simulink model "Constraint"  (R2019a)
settings: Solver=FixedStepAuto  StartTime=0.0  StopTime=100  FixedStep=0.01  RelTol=1e-3
settings Model: Creator=huic  LastModifiedBy=huic
settings SolverCC: MaxConsecutiveZCs=2048

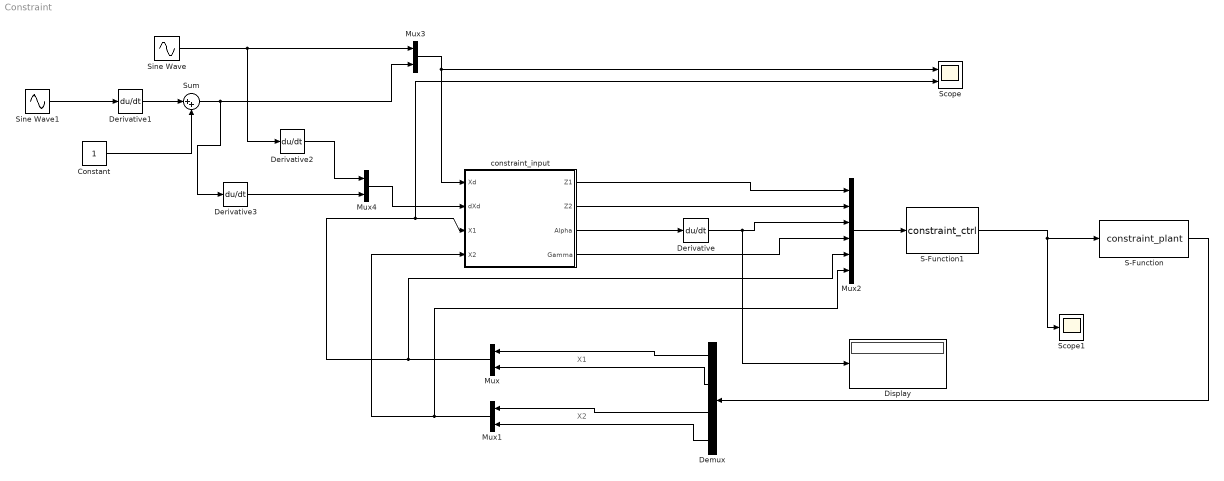
== system Constraint ==
  note: X1
  note: X2
  Constant : Constant
  Demux : Demux
  Derivative{,1..3} (4 alike) : Derivative
  Display : Display
  Mux{,1,3..4} (4 alike) : Mux  Inputs=2
  Mux2 : Mux  Inputs=6
  S-Function : S-Function  FunctionName=constraint_plant  SFunctionDeploymentMode=off  EnableBusSupport=off
  S-Function1 : S-Function  FunctionName=constraint_ctrl  SFunctionDeploymentMode=off  EnableBusSupport=off
  Scope : Scope  NumInputPorts=2
  Scope1 : Scope
  Sine Wave : Sin  SampleTime=0
  Sine Wave1 : Sin  Amplitude=0.3  SampleTime=0
  Sum : Sum  Inputs=|++
  constraint_input : MATLAB Function  TreatAsAtomicUnit=on
  wires:
  S-Function/1 -> Demux/1
  Demux/1 -> Mux/1
  Mux/1 -> Mux2/5, Scope/2, constraint_input/3(X1)
  Demux/4 -> Mux1/2
  Mux1/1 -> Mux2/6, constraint_input/4(X2)
  Demux/2 -> Mux/2
  Demux/3 -> Mux1/1
  constraint_input/1(Z1) -> Mux2/1
  constraint_input/2(Z2) -> Mux2/2
  constraint_input/3(Alpha) -> Derivative/1
  Derivative/1 -> Display/1, Mux2/3
  constraint_input/4(Gamma) -> Mux2/4
  Mux2/1 -> S-Function1/1
  S-Function1/1 -> Scope1/1, S-Function/1
  Sine Wave/1 -> Derivative2/1, Mux3/1
  Sine Wave1/1 -> Derivative1/1
  Derivative1/1 -> Sum/1
  Constant/1 -> Sum/2
  Sum/1 -> Derivative3/1, Mux3/2
  Mux3/1 -> Scope/1, constraint_input/1(Xd)
  Mux4/1 -> constraint_input/2(dXd)
  Derivative2/1 -> Mux4/1
  Derivative3/1 -> Mux4/2

== matlab function Constraint/constraint_input ==
  data: Xd input; dXd input; X1 input; Z1 output; X2 input; Z2 output; Alpha output; Gamma output
function [Z1,Z2,Alpha,Gamma] = constraint_input(Xd,dXd,X1,X2)
up_delat = [1.1;1.35];    %关节1和关节2的上下限
low_delat = [-1.2;0.2];
A=(up_delat - low_delat)./2;  %A和B为转换系数
B=(up_delat + low_delat)./2;
C1=diag([12 10]);

sd1=tan((Xd(1)-B(1))/A(1));
sd2=tan((Xd(2)-B(2))/A(2));
Sd=[sd1;sd2];

s1=tan((X1(1)-B(1))/A(1));
s2=tan((X1(2)-B(2))/A(2));
S1=[s1;s2];

Z1 = S1-Sd;

%S1的导对应的gamma
gamma1 = 1/A(1)*(1+s1*s1);
gamma2 = 1/A(2)*(1+s2*s2);
gamma = [gamma1;gamma2];
% ds11=gamma1*X2(1); 
% ds12=gamma2*X2(2);
% dS1=[ds11;ds12];

%Sd的导对应的gamma
gamma1_d = 1/A(1)*(1+sd1*sd1);
gamma2_d = 1/A(2)*(1+sd2*sd2);



dsd1=gamma1_d*dXd(1);
dsd2=gamma2_d*dXd(2);
dSd=[dsd1;dsd2];

alpha11=-(C1(1,1)/gamma1+1/4*gamma1)*Z1(1)+dSd(1)/gamma1;
alpha12=-(C1(2,2)/gamma2+1/4*gamma2)*Z1(2)+dSd(2)/gamma2;
alpha1=[alpha11;alpha12];

Z2=X2-alpha1;
Alpha = alpha1;
Gamma = gamma;
